simulink model "FunctionCallSS1"  (R2017b)
settings: Solver=FixedStepDiscrete  StartTime=0.0  StopTime=19.8  FixedStep=0.200000  RelTol=1e-3
libraries: simulink x1
settings Model: Creator=hbourbou  LastModifiedBy=hbourbou
settings DataIOCC: ExternalInput=input_dataset  LoadExternalInput=on  SaveState=on
settings DebuggingCC: AlgebraicLoopMsg=error
settings GRTTargetCC: ExtMode=on

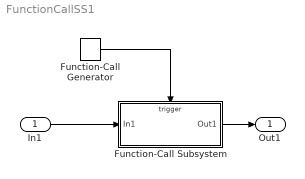
== system FunctionCallSS1 ==
  In1 : Inport
  Function-Call Generator : simulink/Ports & Subsystems/Function-Call Generator  sample_time=1  numberOfIterations=1
  Function-Call Subsystem : Subsystem  TreatAsAtomicUnit=on
  Out1 : Outport
  wires:
  In1/1 -> Function-Call Subsystem/1(In1)
  Function-Call Subsystem/1(Out1) -> Out1/1
  Function-Call Generator/1 -> Function-Call Subsystem/Trigger

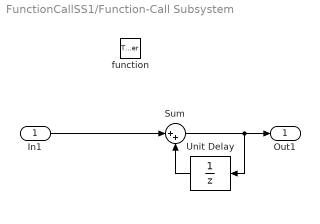
== system FunctionCallSS1/Function-Call Subsystem ==
  In1 : Inport
  function : TriggerPort  TriggerType=function-call  VariantControl=Variant
  Sum : Sum  Inputs=|++
  Unit Delay : UnitDelay  SampleTime=-1
  Out1 : Outport
  wires:
  In1/1 -> Sum/1
  Sum/1 -> Unit Delay/1, Out1/1
  Unit Delay/1 -> Sum/2
